simulink model "coeff_estimation"  (R2018a)
settings: Solver=FixedStepDiscrete  StartTime=0.0  StopTime=10  RelTol=1e-3  EnableMultiTasking=on
libraries: audiosources x1, dspsnks4 x1, dspsrcs4 x1
settings Model: Creator=gianc  LastModifiedBy=gianc

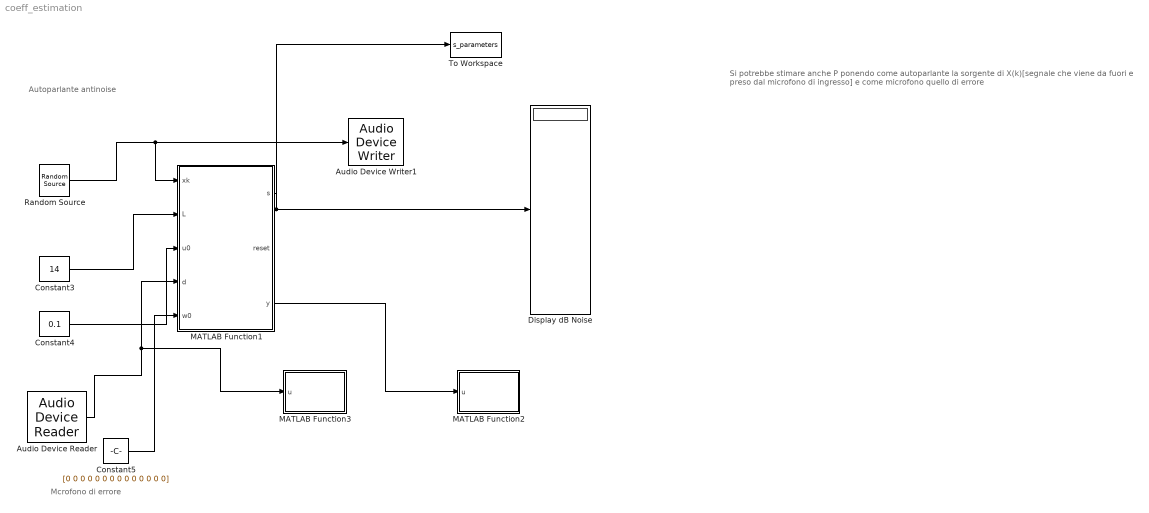
== system coeff_estimation ==
  note: Autoparlante antinoise
  note: Si potrebbe stimare anche P ponendo come autoparlante la sorgente di X(k)[segnale che viene da fuori e preso dal microfono di ingresso] e come microfono quello di errore
  note: Mcrofono di errore
  Audio Device Reader : audiosources/Audio Device Reader  Driver=DirectSound  Device=Microfono (2- USB PnP Sound Device)  SampleRate=8000  NumChannels=1  SamplesPerFrame=255  BitDepth=16-bit integer  NumBuffers=10  DefaultInputChannelMapping=on  InputChannelMapping=1:2  OutputNumOverrunSamples=off  OutputDataType=double  DriverIdx=1  DeviceWarnFlag=''
      settings: SourceProductName=Audio System Toolbox  SourceProductBaseCode=AU
  Audio Device Writer1 : dspsnks4/Audio Device Writer  Driver=DirectSound  Device=Default  InheritSampleRate=off  SampleRate=8000  BitDepth=16-bit integer  BufferSize=4096  NumBuffers=10  DefaultOutputChannelMapping=on  OutputChannelMapping=1:2  OutputNumUnderrunSamples=off  DriverIdx=1  DeviceWarnFlag=''
  Constant3 : Constant  Value=14
  Constant4 : Constant  Value=0.1
  Constant5 : Constant  Value=[0 0 0 0 0 0 0 0 0 0 0 0 0 0]  VectorParams1D=off
  Display dB Noise : Display
  MATLAB Function1 : MATLAB Function  TreatAsAtomicUnit=on
  MATLAB Function2 : MATLAB Function  TreatAsAtomicUnit=on
  MATLAB Function3 : MATLAB Function  TreatAsAtomicUnit=on
  Random Source : dspsrcs4/Random Source  SrcType=Uniform  NormMethod=Ziggurat  CltLength=12  MinVal=0  MaxVal=3  MeanVal=0  VarVal=1  RepMode=Not repeatable  rawSeed=1  IsInherit=off  SampMode=Discrete  SampTime=1/8000  SampFrame=255  DataType=Double  OutComplex=Real  OutputFrames=off
  To Workspace : ToWorkspace  VariableName=s_parameters  SampleTime=-1
      settings: MaxDataPoints=1  Save2DSignal=2-D array (concatenate along first dimension)
  wires:
  Constant4/1 -> MATLAB Function1/3(u0)
  Constant3/1 -> MATLAB Function1/2(L)
  Constant5/1 -> MATLAB Function1/5(w0)
  Random Source/1 -> MATLAB Function1/1(xk), Audio Device Writer1/1
  Audio Device Reader/1 -> MATLAB Function3/1(u), MATLAB Function1/4(d)
  MATLAB Function1/1(s) -> To Workspace/1, Display dB Noise/1
  MATLAB Function1/3(y) -> MATLAB Function2/1(u)

== matlab function coeff_estimation/MATLAB Function1 ==
  data: s output; xk input; L input; u0 input; d input; reset output; w0 input; y output
%y=output filter (anti noise)
%w=weights vector 1xL
%x=input vector 1xL
%xk=sampled input at time k
%d=wanted signal (ideal is x but we have d=P*x)

function [s,reset,y] = LMS_estimation(xk,L,u0,d,w0)

%global variables
[sizeD,~]=size(xk);
y=zeros(sizeD,1);
e=zeros(sizeD,1);
u=u0;
alpha=0.6;
persistent cnt
persistent x
persistent w
persistent r

for i=1:sizeD
    
if isempty(cnt)
    cnt=1;
else
    cnt=cnt+1;
end

if isempty(x)
    x=zeros(1,L);
end

if isempty(r)
    r=0;
end

if isempty(w)
    w=w0;
end

if cnt<=L
    u=u0;
else
    if cnt==L
        u = alpha/(x*(x'));
    else
        u = alpha/max(u/alpha,x*(x'));
    end
end
u
x=[xk(i,1) x(1:(L-1))]; %shift and add xk (FIFO)
y(i)= w*(x');
e(i)= d(i)- y(i);
w = w + u*x*e(i); %refresh w for the next iteration
end
s=w;
reset=r;
end

== matlab function coeff_estimation/MATLAB Function2 ==
  data: u input
function fcn(u)
persistent t
if isempty(t)
    t=ones(255,1);
else
    t(1)=t(255)+1;
end

for i=1:254
    t(i+1)=t(i)+1;
end

hold on
plot(t,u,'g');

end

== matlab function coeff_estimation/MATLAB Function3 ==
  data: u input
function fcn(u)
persistent t
if isempty(t)
    t=ones(255,1);
else
    t(1)=t(255)+1;
end

for i=1:254
    t(i+1)=t(i)+1;
end

hold on
plot(t,u,'b');

end
